simulink model "simulink_posta_1"  (R2021a)
settings: Solver=VariableStepAuto  StartTime=0.0  StopTime=10000  FixedStep=0.1  RelTol=1e-3
undefined symbols (not defined in the file): Earth, WGS84
libraries: aerolib6dof2 x1, sharedtransform x1
settings Model: Creator=Euge Etcheverry  LastModifiedBy=Fabricio

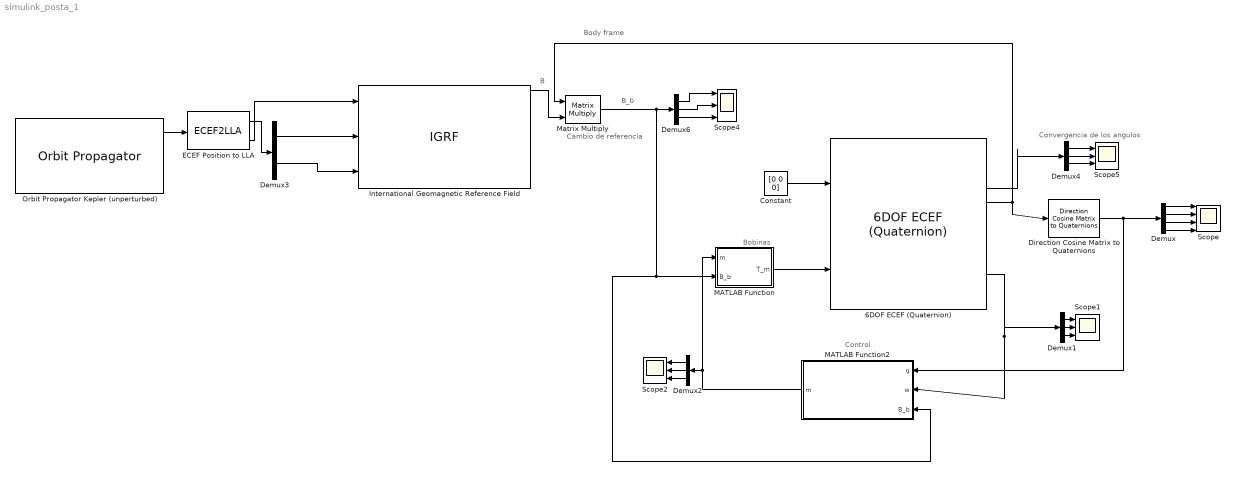
== system simulink_posta_1 ==
  note: Control
  note: Bobinas
  note: Body frame
  note: B
  note: B_b
  note: Cambio de referencia
  note: Convergencia de los angulos
  6DOF ECEF (Quaternion) : aerolib6dof2/6DOF ECEF (Quaternion)  units=Metric (MKS)  mtype=Fixed  xg_0=[0 0 0]  Vm_0=[0 0 0]  eul_0=[0.1 0.5 0.5]  pm_0=[1 1 1]*pi/180  mass_0=1.0  mass_e=0.5  mass_f=2.0  inertia=2e-3*eye(3)  inertia_e=eye(3)  inertia_f=2*eye(3)  vre_flag=on  abi_flag=off  ptype=Earth (WGS84)  R=6378137  F=1/298.257223563  w_E=7292115e-11  angle_in=Internal  LG0=0  quat_statename=''  pm_statename=''  Vm_statename=''  posECEF_statename=''  posECI_statename=''  LG_statename=''  mass_statename=''
      settings: SourceProductBaseCode=AE
  Constant : Constant  Value=[0 0 0]
  Demux : Demux
  Demux{1..2,4,6} (4 alike) : Demux  Outputs=3
  Demux3 : Demux  Outputs=2
  Direction Cosine Matrix to Quaternions : sharedtransform/Direction Cosine Matrix  to Quaternions  aMode=0  action=None  tolerance=eps(2)
      settings: SourceProductBaseCode=AE,PW,DR,MT,UV,VE
  ECEF Position to LLA : ECEF2LLA
  International Geomagnetic Reference Field : IGRF  time_in=off  month=February  day=23  year=2024
      settings: AttributesFormatString=%<generation>
  MATLAB Function : MATLAB Function  TreatAsAtomicUnit=on
  MATLAB Function2 : MATLAB Function  TreatAsAtomicUnit=on  SystemSampleTime=1e-3
  Matrix Multiply : Product  Multiplication=Matrix(*)
  Orbit Propagator Kepler (unperturbed) : OrbitPropagator  startDate=[2024, 02, 23, 12, 32, 16]  eccentricity=0.0005  inclination=98.06  raan=105  trueAnomaly=180  customMu=4.305e13  customJ2=1.0826269e-03  timeFormat=Gregorian
  Scope : Scope  NumInputPorts=4
  Scope{1..2,4..5} (4 alike) : Scope  NumInputPorts=3
  wires:
  6DOF ECEF (Quaternion)/5 -> Direction Cosine Matrix to Quaternions/1, Matrix Multiply/1
  Direction Cosine Matrix to Quaternions/1 -> MATLAB Function2/1(q), Demux/1
  Demux/1 -> Scope/1
  Demux/3 -> Scope/3
  Demux/4 -> Scope/4
  Demux/2 -> Scope/2
  Demux4/1 -> Scope5/1
  Demux4/2 -> Scope5/2
  Demux4/3 -> Scope5/3
  6DOF ECEF (Quaternion)/4 -> Demux4/1
  ECEF Position to LLA/1 -> Demux3/1
  Orbit Propagator Kepler (unperturbed)/1 -> ECEF Position to LLA/1
  International Geomagnetic Reference Field/1 -> Matrix Multiply/2
  Matrix Multiply/1 -> MATLAB Function2/3(B_b), MATLAB Function/2(B_b), Demux6/1
  Constant/1 -> 6DOF ECEF (Quaternion)/1
  Demux6/1 -> Scope4/1
  Demux6/2 -> Scope4/2
  Demux6/3 -> Scope4/3
  ECEF Position to LLA/2 -> International Geomagnetic Reference Field/1
  Demux3/1 -> International Geomagnetic Reference Field/2
  Demux3/2 -> International Geomagnetic Reference Field/3
  MATLAB Function2/1(m) -> Demux2/1, MATLAB Function/1(m)
  6DOF ECEF (Quaternion)/10 -> Demux1/1, MATLAB Function2/2(w)
  Demux1/1 -> Scope1/1
  Demux1/2 -> Scope1/2
  Demux1/3 -> Scope1/3
  Demux2/1 -> Scope2/1
  Demux2/2 -> Scope2/2
  Demux2/3 -> Scope2/3
  MATLAB Function/1(T_m) -> 6DOF ECEF (Quaternion)/2

== matlab function simulink_posta_1/MATLAB Function ==
  data: m input; T_m output; B_b input
function T_m = fcn(m, B_b)

%saturacion; Tener en cuenta que pueden ser diferentes
top = [0.1, 0.1, 0.1]';
m_res = [45e-4, 45e-4, 45e-4]';

for i=1:3
    if abs(m(i)) > top(i)
        m(i) = sign(m(i))*top(i);
    end
end

T_m = cross(m + m_res*0, B_b*1e-9);

== matlab function simulink_posta_1/MATLAB Function2 ==
  data: q input; m output; w input; B_b input
function m = fcn(q, w, B_b)


q0 = q(1);
q = q(2:4);

epsilon = 0.001;


K = 2e-3*eye(3)*20; %alpha*J/Jmax
w_M = 0.01;

u = -epsilon*K*w;

persistent sgn_q0;
persistent kq;
kq = 0;
if isempty(sgn_q0)
    if  norm(w) < w_M
        sgn_q0 = sign(q0);
    end
else
    kq = 0.001;
    u = -epsilon*epsilon*kq*sgn_q0*q + u;
end

m = cross(B_b*1e-9,u)/(norm(B_b*1e-9).^2);
